simulink model "Chou"  (Simulink 2.20)
settings: Solver=ode45  StartTime=0.0  StopTime=9999  MaxStep=0.001  RelTol=1e-5  AbsTol=1e-5
settings Model: SaveTime=off  SaveOutput=off  ConsistencyChecking=off  RTWPlaceOutputsASAP=off

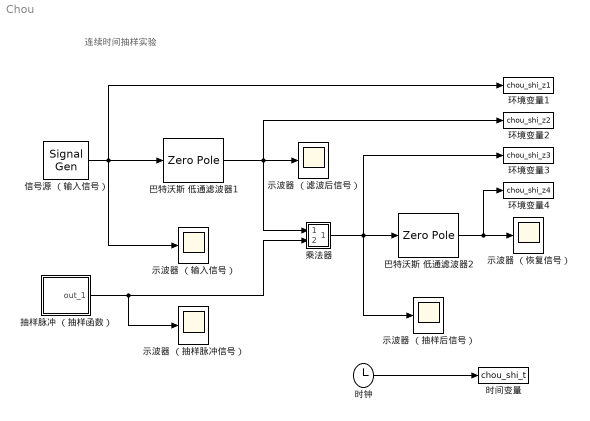
== system Chou ==
  note: 连续时间抽样实验
  巴特沃斯 低通滤波器1 : ZeroPole  Zeros=z  Poles=p  Gain=k  mask(buttap){@1=60, @2=4}
      mask prompts: @1 "Cutoff frequency (rad/sec)"; @2 "Order"
      mask help:
      | Analog Butterworth low pass filter.
      |
      | (Requires Signal Processing Toolbox)
      mask init:
      | [z,p,k]=buttap(@2); z=@1*z; p=@1*p; k=real(prod(-p)); [num,den]=zp2tf(z,p,k); w=logspace(log10(@1/10),log10(10*@1),20); h=freqs(num,den,w);
      mask Help: Butterworth low pass filter using MATLAB's butter command.
      mask Display: plot(20*log10(w),20*log10(abs(h)))
  巴特沃斯 低通滤波器2 : ZeroPole  Zeros=z  Poles=p  Gain=k  mask(buttap){@1=60, @2=4}
      mask prompts: @1 "Cutoff frequency (rad/sec)"; @2 "Order"
      mask help:
      | Analog Butterworth low pass filter.
      |
      | (Requires Signal Processing Toolbox)
      mask init:
      | [z,p,k]=buttap(@2); z=@1*z; p=@1*p; k=real(prod(-p)); [num,den]=zp2tf(z,p,k); w=logspace(log10(@1/10),log10(10*@1),20); h=freqs(num,den,w);
      mask Help: Butterworth low pass filter using MATLAB's butter command.
      mask Display: plot(20*log10(w),20*log10(abs(h)))
  乘法器 : Subsystem
      mask Type: Dot Product
      mask Description:
      | Inner (dot) product.
      | y=sum(u1.*u2)
      mask Help: Computes the inner (dot) product of the inputs: sum(u1.*u2).  The inputs are vectors of the same length. Output is a scalar.
      mask Display: disp('X')
  抽样脉冲 （抽样函数） : Subsystem  mask(Pulse Generator){@1=pi/100, @2=0.001, @3=5, @4=0.0005}
      mask prompts: @1 "Pulse period (secs):"; @2 "Pulse width:"; @3 "Pulse height:"; @4 "Pulse start time:"
      mask help: Pulse Generator.
      mask init:
      | Ts=@1; du=@2; ht=@3; stt=@4; ini=ones(length(ht),1); st1=rem(stt,Ts); st2=rem(stt+du,Ts);if(Ts<=1.2*du),ini=zeros(length(ht),1);end;
      mask Help: Pulse generator which ensures pulse\ntransitions are hit. Provides a vector of pulses when the height is entered as a vector.\nUnmask to see how it works.
      mask Display: plot(0,0,100,100,[90,75,75,60,60,35,35,20,20,10],[20,20,80,80,20,20,80,80,20,20])
  环境变量1 : ToWorkspace  VariableName=chou_shi_z1  SampleTime=0.001
      settings: Buffer=4096
  环境变量2 : ToWorkspace  VariableName=chou_shi_z2  SampleTime=0.001
      settings: Buffer=4096
  环境变量3 : ToWorkspace  VariableName=chou_shi_z3  SampleTime=0.001
      settings: Buffer=4096
  环境变量4 : ToWorkspace  VariableName=chou_shi_z4  SampleTime=0.001
      settings: Buffer=4096
  "时间变量 " : ToWorkspace  VariableName=chou_shi_t  SampleTime=0.001
      settings: Buffer=4096
  "时钟 " : Clock
  示波器 （抽样后信号） : Scope
      settings: TickLabels=on  TimeRange=3.000000  YMin=-14  YMax=14  SaveToWorkspace=off  SaveName=ScopeData
  示波器 （抽样脉冲信号） : Scope
      settings: TickLabels=on  TimeRange=1.000000  YMin=-8  YMax=8  SaveToWorkspace=off  SaveName=ScopeData
  示波器 （恢复信号） : Scope
      settings: TickLabels=on  TimeRange=3.000000  YMin=-1  YMax=1  SaveToWorkspace=off  SaveName=ScopeData
  "示波器 （滤波后信号） " : Scope
      settings: TickLabels=on  TimeRange=3.000000  YMin=-4  YMax=4  SaveToWorkspace=off  SaveName=ScopeData
  示波器 （输入信号） : Scope
      settings: TickLabels=on  TimeRange=3.000000  YMin=-4.000000  YMax=4.000000  SaveToWorkspace=off  SaveName=ScopeData
  "信号源 （输入信号）  " : SignalGenerator  WaveForm=sine  Amplitude=2.000000  Frequency=6.000000  Units=rad/sec
  wires:
  乘法器/1(out_1) -> 巴特沃斯 低通滤波器2/1, 示波器 （抽样后信号）/1, 环境变量3/1
  抽样脉冲 （抽样函数）/1(out_1) -> 乘法器/2(in_2), 示波器 （抽样脉冲信号）/1
  巴特沃斯 低通滤波器2/1 -> 示波器 （恢复信号）/1, 环境变量4/1
  "时钟 "/1 -> "时间变量 "/1
  "信号源 （输入信号）  "/1 -> 示波器 （输入信号）/1, 环境变量1/1, 巴特沃斯 低通滤波器1/1
  巴特沃斯 低通滤波器1/1 -> 乘法器/1(in_1), "示波器 （滤波后信号） "/1, 环境变量2/1

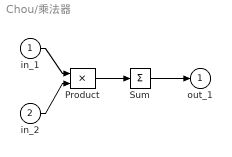
== system Chou/乘法器 ==
  in_1 : Inport  Port=1  PortWidth=-1  SampleTime=-1
  in_2 : Inport  Port=2  PortWidth=-1  SampleTime=-1
  Product : Product  Inputs=2
  Sum : Sum  Inputs=+
  out_1 : Outport  Port=1
  wires:
  in_2/1 -> Product/2
  in_1/1 -> Product/1
  Product/1 -> Sum/1
  Sum/1 -> out_1/1

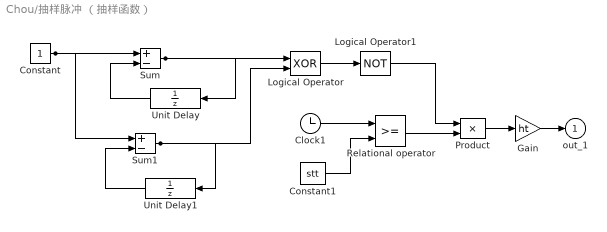
== system Chou/抽样脉冲 （抽样函数） ==
  Clock1 : Clock
  Constant : Constant  Value=1
  Constant1 : Constant  Value=stt
  Gain : Gain  Gain=ht
  Logical Operator : Logic  Operator=XOR  Inputs=2
  Logical Operator1 : Logic  Operator=NOT  Inputs=1
  Product : Product  Inputs=2
  Relational operator : RelationalOperator  Operator=>=
  Sum : Sum  Inputs=+-
  Sum1 : Sum  Inputs=+-
  Unit Delay : UnitDelay  Orientation=left  X0=0  SampleTime=[Ts,st1]
  Unit Delay1 : UnitDelay  Orientation=left  X0=ini  SampleTime=[Ts,st2]
  out_1 : Outport  Port=1
  wires:
  Logical Operator1/1 -> Product/1
  Logical Operator/1 -> Logical Operator1/1
  Constant1/1 -> Relational operator/2
  Gain/1 -> out_1/1
  Product/1 -> Gain/1
  Relational operator/1 -> Product/2
  Clock1/1 -> Relational operator/1
  Unit Delay/1 -> Sum/2
  Unit Delay1/1 -> Sum1/2
  Constant/1 -> Sum/1, Sum1/1
  Sum/1 -> Unit Delay/1, Logical Operator/1
  Sum1/1 -> Unit Delay1/1, Logical Operator/2
